simulink model "MOSFET_2L_VSI_SPWM_DDsystem"  (R2023a)
settings: Solver=VariableStepAuto  StartTime=0.0  StopTime=simu.endTime  MaxStep=simu.dt  RelTol=1e-3
undefined symbols (not defined in the file): conv, dev
libraries: WECSim_Lib_PTOSim x2
Description:
  | To be used with Wec-Sim's "Direct Drive Linear Generator" Block. Generator parameters MUST match what was set for simulating the WEC with the associated PTO.
settings Model: Creator=bartonsa  LastModifiedBy=bartonsa

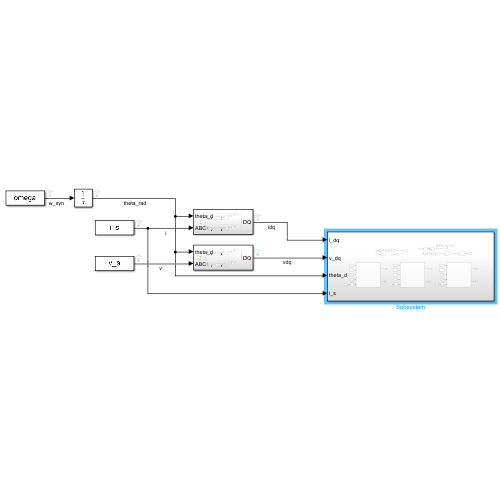
[thumbnail: Simulink's stored preview of the top-level diagram]
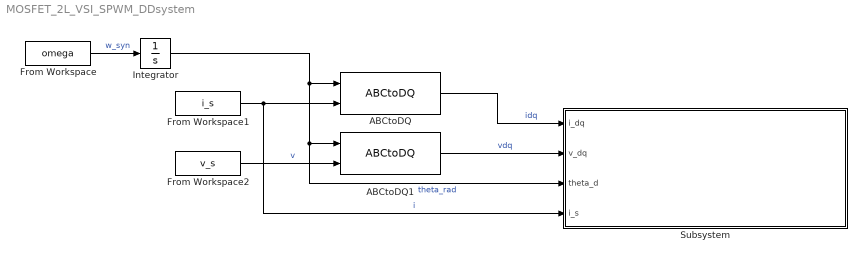
== system MOSFET_2L_VSI_SPWM_DDsystem ==
  ABCtoDQ : WECSim_Lib_PTOSim/Electric/Direct Drive Linear Generator/ABCtoDQ  SystemSampleTime=-1  VariantActivationTime=update diagram  Latency=0  AutoFrameSizeCalculation=off
  ABCtoDQ1 : WECSim_Lib_PTOSim/Electric/Direct Drive Linear Generator/ABCtoDQ  SystemSampleTime=-1  VariantActivationTime=update diagram  Latency=0  AutoFrameSizeCalculation=off
  From Workspace : FromWorkspace  VariableName=omega
  From Workspace1 : FromWorkspace  VariableName=i_s
  From Workspace2 : FromWorkspace  VariableName=v_s
  Integrator : Integrator  WrappedStateLowerValue=0
  Subsystem : Subsystem
  wires:
  ABCtoDQ/1 -> Subsystem/1(i_dq)  "idq"
  ABCtoDQ1/1 -> Subsystem/2(v_dq)  "vdq"
  From Workspace/1 -> Integrator/1  "w_syn"
  Integrator/1 -> Subsystem/3(theta_d), ABCtoDQ1/1, ABCtoDQ/1  "theta_rad"
  From Workspace1/1 -> Subsystem/4(i_s), ABCtoDQ/2  "i"
  From Workspace2/1 -> ABCtoDQ1/2  "v"

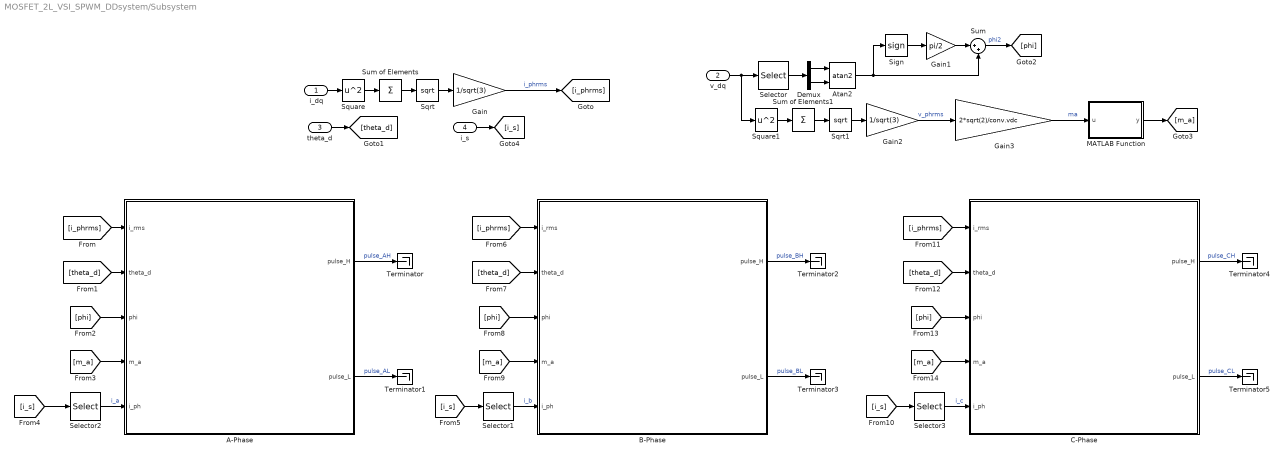
== system MOSFET_2L_VSI_SPWM_DDsystem/Subsystem ==
  i_dq : Inport
  v_dq : Inport  Port=2
  theta_d : Inport  Port=3
  i_s : Inport  Port=4
  A-Phase : Subsystem  AncestorBlock=MPModeling_MOSFETConv_lib/MOSFET 2L VSC/Device 1
      settings: LibrarySourceBlock=MPModeling_MOSFETConv_lib/MOSFET 2L VSC/Device 1
  Atan2 : Trigonometry  Operator=atan2
  B-Phase : Subsystem  AncestorBlock=MPModeling_MOSFETConv_lib/MOSFET 2L VSC/Device 1
      settings: LibrarySourceBlock=MPModeling_MOSFETConv_lib/MOSFET 2L VSC/Device 1
  C-Phase : Subsystem  AncestorBlock=MPModeling_MOSFETConv_lib/MOSFET 2L VSC/Device 1
      settings: LibrarySourceBlock=MPModeling_MOSFETConv_lib/MOSFET 2L VSC/Device 1
  Demux : Demux  Outputs=2
  Gain : Gain  Gain=1/sqrt(3)
  Gain1 : Gain  Gain=pi/2
  Gain2 : Gain  Gain=1/sqrt(3)
  Gain3 : Gain  Gain=2*sqrt(2)/conv.vdc
  MATLAB Function : MATLAB Function  TreatAsAtomicUnit=on
  Selector : Selector  InputPortWidth=2  IndexOptions=Index vector (dialog)  Indices=[2 1]  OutputSizes=1
  Selector1 : Selector  InputPortWidth=3  IndexOptions=Index vector (dialog)  Indices=2  OutputSizes=1
  Selector2 : Selector  InputPortWidth=3  IndexOptions=Index vector (dialog)  Indices=1  OutputSizes=1
  Selector3 : Selector  InputPortWidth=3  IndexOptions=Index vector (dialog)  Indices=3  OutputSizes=1
  Sign : Signum
  Sqrt : Sqrt
  Sqrt1 : Sqrt
  Square : Math  Operator=square
  Square1 : Math  Operator=square
  Sum : Sum  Inputs=|++
  Sum of Elements : Sum  Inputs=+
  Sum of Elements1 : Sum  Inputs=+
  Terminator{,1..5} (6 alike) : Terminator
  wires:
  Sum of Elements/1 -> Sqrt/1
  v_dq/1 -> Selector/1, Square1/1
  Gain/1 -> [i_phrms]  "i_phrms"
  i_dq/1 -> Square/1
  Square/1 -> Sum of Elements/1
  theta_d/1 -> [theta_d]
  Selector/1 -> Demux/1
  Sqrt/1 -> Gain/1
  A-Phase/1(pulse_H) -> Terminator/1  "pulse_AH"
  Demux/1 -> Atan2/1
  Demux/2 -> Atan2/2
  Atan2/1 -> Sum/2, Sign/1
  Square1/1 -> Sum of Elements1/1
  Sqrt1/1 -> Gain2/1
  Sum of Elements1/1 -> Sqrt1/1
  Gain2/1 -> Gain3/1  "v_phrms"
  Gain3/1 -> MATLAB Function/1(u)  "ma"
  i_s/1 -> [i_s]
  Selector2/1 -> A-Phase/5(i_ph)  "i_a"
  A-Phase/2(pulse_L) -> Terminator1/1  "pulse_AL"
  [i_phrms] -> A-Phase/1(i_rms)
  [theta_d] -> A-Phase/2(theta_d)
  [phi] -> A-Phase/3(phi)
  [m_a] -> A-Phase/4(m_a)
  [i_s] -> Selector2/1
  Selector1/1 -> B-Phase/5(i_ph)  "i_b"
  [i_s] -> Selector1/1
  [i_phrms] -> B-Phase/1(i_rms)
  [theta_d] -> B-Phase/2(theta_d)
  [phi] -> B-Phase/3(phi)
  [m_a] -> B-Phase/4(m_a)
  B-Phase/2(pulse_L) -> Terminator3/1  "pulse_BL"
  B-Phase/1(pulse_H) -> Terminator2/1  "pulse_BH"
  [phi] -> C-Phase/3(phi)
  C-Phase/2(pulse_L) -> Terminator5/1  "pulse_CL"
  [theta_d] -> C-Phase/2(theta_d)
  [i_phrms] -> C-Phase/1(i_rms)
  C-Phase/1(pulse_H) -> Terminator4/1  "pulse_CH"
  Selector3/1 -> C-Phase/5(i_ph)  "i_c"
  [i_s] -> Selector3/1
  [m_a] -> C-Phase/4(m_a)
  MATLAB Function/1(y) -> [m_a]
  Sign/1 -> Gain1/1
  Gain1/1 -> Sum/1
  Sum/1 -> [phi]  "phi2"

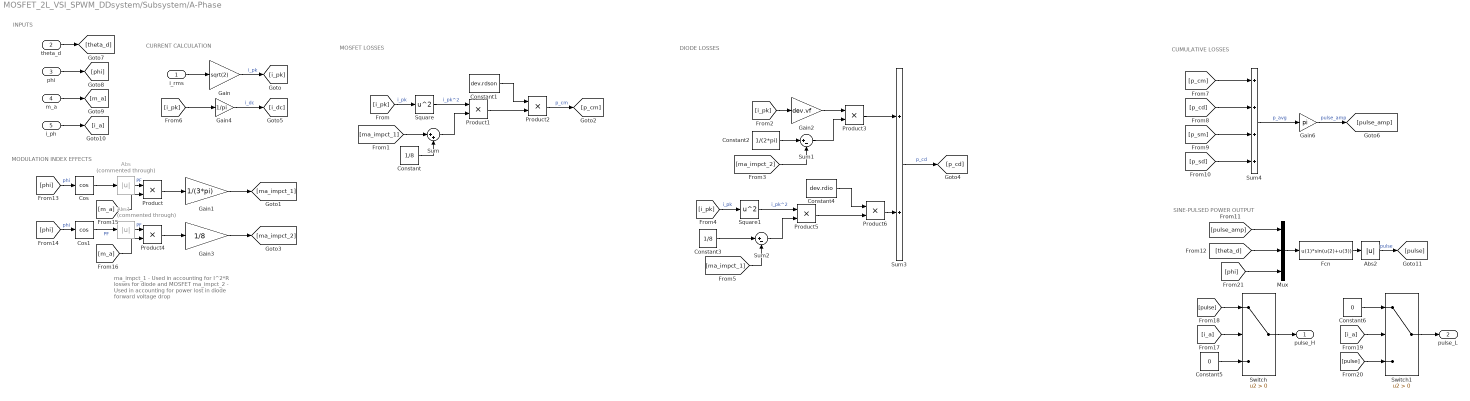
== system MOSFET_2L_VSI_SPWM_DDsystem/Subsystem/A-Phase ==
  note: INPUTS
  note: CURRENT CALCULATION
  note: SINE-PULSED POWER OUTPUT
  note: MODULATION INDEX EFFECTS
  note: ma_impct_1 - Used in accounting for I^2*R losses for diode and MOSFET
      |
      | ma_impct_2 - Used in accounting for power lost in diode forward voltage drop
  note: MOSFET LOSSES
  note: DIODE LOSSES
  note: CUMULATIVE LOSSES
  i_rms : Inport
  theta_d : Inport  Port=2
  phi : Inport  Port=3
  m_a : Inport  Port=4
  i_ph : Inport  Port=5
  Abs : Abs  Commented=through  SaturateOnIntegerOverflow=off
  Abs1 : Abs  Commented=through  SaturateOnIntegerOverflow=off
  Abs2 : Abs  SaturateOnIntegerOverflow=off
  Constant : Constant  Value=1/8
  Constant1 : Constant  Value=dev.rdson
  Constant2 : Constant  Value=1/(2*pi)
  Constant3 : Constant  Value=1/8
  Constant4 : Constant  Value=dev.rdio
  Constant5 : Constant  Value=0
  Constant6 : Constant  Value=0
  Cos : Trigonometry  Operator=cos
  Cos1 : Trigonometry  Operator=cos
  Fcn : Fcn  Expr=u(1)*sin(u(2)+u(3))
  Gain : Gain  Gain=sqrt(2)
  Gain1 : Gain  Gain=1/(3*pi)
  Gain2 : Gain  Gain=dev.vf
  Gain3 : Gain  Gain=1/8
  Gain4 : Gain  Gain=1/pi
  Gain6 : Gain  Gain=pi
  Mux : Mux  Inputs=3
  Product{,1..6} (7 alike) : Product
  Square : Math  Operator=square
  Square1 : Math  Operator=square
  Sum : Sum  Inputs=|++
  Sum1 : Sum  Inputs=|+-
  Sum2 : Sum  Inputs=|+-
  Sum3 : Sum
  Sum4 : Sum  Inputs=++++
  Switch : Switch  Criteria=u2 > Threshold  SaturateOnIntegerOverflow=off  InputSameDT=off
  Switch1 : Switch  Criteria=u2 > Threshold  SaturateOnIntegerOverflow=off  InputSameDT=off
  pulse_H : Outport
  pulse_L : Outport  Port=2
  wires:
  Mux/1 -> Fcn/1
  m_a/1 -> [m_a]
  phi/1 -> [phi]
  Abs2/1 -> [pulse]  "pulse"
  theta_d/1 -> [theta_d]
  [phi] -> Cos/1  "phi"
  Sum2/1 -> Product5/2
  [ma_impct_1] -> Sum2/2
  Constant3/1 -> Sum2/1
  Square1/1 -> Product5/1  "i_pk^2"
  Constant2/1 -> Sum1/1
  Gain2/1 -> Product3/1
  Cos1/1 -> Abs1/1  "PF"
  Gain3/1 -> [ma_impct_2]
  [ma_impct_1] -> Sum/1
  Fcn/1 -> Abs2/1
  Sum4/1 -> Gain6/1  "p_avg"
  [p_sd] -> Sum4/4
  Product6/1 -> Sum3/2
  [p_cm] -> Sum4/1
  [p_cd] -> Sum4/2
  [phi] -> Cos1/1  "phi"
  Gain4/1 -> [i_dc]  "i_dc"
  Constant4/1 -> Product6/1
  [i_pk] -> Gain2/1
  Constant1/1 -> Product2/1
  Product3/1 -> Sum3/1
  [i_pk] -> Gain4/1
  Product2/1 -> [p_cm]  "p_cm"
  Product4/1 -> Gain3/1
  Sum1/1 -> Product3/2
  i_rms/1 -> Gain/1
  [ma_impct_2] -> Sum1/2
  Square/1 -> Product1/1  "i_pk^2"
  Constant/1 -> Sum/2
  Gain/1 -> [i_pk]  "i_pk"
  [i_pk] -> Square1/1  "i_pk"
  Product5/1 -> Product6/2
  Cos/1 -> Abs/1
  Product1/1 -> Product2/2
  Sum3/1 -> [p_cd]  "p_cd"
  [i_pk] -> Square/1  "i_pk"
  Gain1/1 -> [ma_impct_1]
  [p_sm] -> Sum4/3
  [pulse_amp] -> Mux/1
  Sum/1 -> Product1/2
  Product/1 -> Gain1/1
  Abs/1 -> Product/1  "PF"
  Abs1/1 -> Product4/1  "PF"
  [m_a] -> Product/2
  [m_a] -> Product4/2
  [theta_d] -> Mux/2
  Switch/1 -> pulse_H/1
  [i_a] -> Switch/2
  Constant5/1 -> Switch/3
  Gain6/1 -> [pulse_amp]  "pulse_amp"
  i_ph/1 -> [i_a]
  [pulse] -> Switch/1
  Switch1/1 -> pulse_L/1
  [i_a] -> Switch1/2
  Constant6/1 -> Switch1/1
  [pulse] -> Switch1/3
  [phi] -> Mux/3

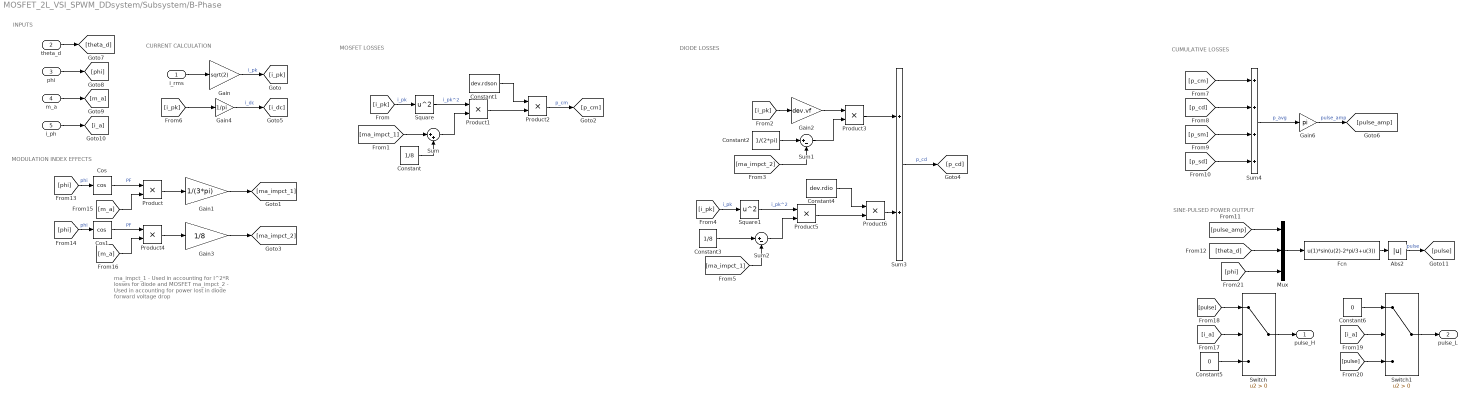
== system MOSFET_2L_VSI_SPWM_DDsystem/Subsystem/B-Phase ==
  note: INPUTS
  note: CURRENT CALCULATION
  note: SINE-PULSED POWER OUTPUT
  note: MODULATION INDEX EFFECTS
  note: ma_impct_1 - Used in accounting for I^2*R losses for diode and MOSFET
      |
      | ma_impct_2 - Used in accounting for power lost in diode forward voltage drop
  note: MOSFET LOSSES
  note: DIODE LOSSES
  note: CUMULATIVE LOSSES
  i_rms : Inport
  theta_d : Inport  Port=2
  phi : Inport  Port=3
  m_a : Inport  Port=4
  i_ph : Inport  Port=5
  Abs2 : Abs  SaturateOnIntegerOverflow=off
  Constant : Constant  Value=1/8
  Constant1 : Constant  Value=dev.rdson
  Constant2 : Constant  Value=1/(2*pi)
  Constant3 : Constant  Value=1/8
  Constant4 : Constant  Value=dev.rdio
  Constant5 : Constant  Value=0
  Constant6 : Constant  Value=0
  Cos : Trigonometry  Operator=cos
  Cos1 : Trigonometry  Operator=cos
  Fcn : Fcn  Expr=u(1)*sin(u(2)-2*pi/3+u(3))
  Gain : Gain  Gain=sqrt(2)
  Gain1 : Gain  Gain=1/(3*pi)
  Gain2 : Gain  Gain=dev.vf
  Gain3 : Gain  Gain=1/8
  Gain4 : Gain  Gain=1/pi
  Gain6 : Gain  Gain=pi
  Mux : Mux  Inputs=3
  Product{,1..6} (7 alike) : Product
  Square : Math  Operator=square
  Square1 : Math  Operator=square
  Sum : Sum  Inputs=|++
  Sum1 : Sum  Inputs=|+-
  Sum2 : Sum  Inputs=|+-
  Sum3 : Sum
  Sum4 : Sum  Inputs=++++
  Switch : Switch  Criteria=u2 > Threshold  SaturateOnIntegerOverflow=off  InputSameDT=off
  Switch1 : Switch  Criteria=u2 > Threshold  SaturateOnIntegerOverflow=off  InputSameDT=off
  pulse_H : Outport
  pulse_L : Outport  Port=2
  wires:
  Mux/1 -> Fcn/1
  m_a/1 -> [m_a]
  phi/1 -> [phi]
  Abs2/1 -> [pulse]  "pulse"
  theta_d/1 -> [theta_d]
  [phi] -> Cos/1  "phi"
  Sum2/1 -> Product5/2
  [ma_impct_1] -> Sum2/2
  Constant3/1 -> Sum2/1
  Square1/1 -> Product5/1  "i_pk^2"
  Constant2/1 -> Sum1/1
  Gain2/1 -> Product3/1
  Gain3/1 -> [ma_impct_2]
  [ma_impct_1] -> Sum/1
  Fcn/1 -> Abs2/1
  Sum4/1 -> Gain6/1  "p_avg"
  [p_sd] -> Sum4/4
  Product6/1 -> Sum3/2
  [p_cm] -> Sum4/1
  [p_cd] -> Sum4/2
  [phi] -> Cos1/1  "phi"
  Gain4/1 -> [i_dc]  "i_dc"
  Constant4/1 -> Product6/1
  [i_pk] -> Gain2/1
  Constant1/1 -> Product2/1
  Product3/1 -> Sum3/1
  [i_pk] -> Gain4/1
  Product2/1 -> [p_cm]  "p_cm"
  Product4/1 -> Gain3/1
  Sum1/1 -> Product3/2
  i_rms/1 -> Gain/1
  [ma_impct_2] -> Sum1/2
  Square/1 -> Product1/1  "i_pk^2"
  Constant/1 -> Sum/2
  Gain/1 -> [i_pk]  "i_pk"
  [i_pk] -> Square1/1  "i_pk"
  Product5/1 -> Product6/2
  Product1/1 -> Product2/2
  Sum3/1 -> [p_cd]  "p_cd"
  [i_pk] -> Square/1  "i_pk"
  Gain1/1 -> [ma_impct_1]
  [p_sm] -> Sum4/3
  [pulse_amp] -> Mux/1
  Sum/1 -> Product1/2
  Product/1 -> Gain1/1
  Cos/1 -> Product/1  "PF"
  Cos1/1 -> Product4/1  "PF"
  [m_a] -> Product/2
  [m_a] -> Product4/2
  [theta_d] -> Mux/2
  Switch/1 -> pulse_H/1
  [i_a] -> Switch/2
  Constant5/1 -> Switch/3
  Gain6/1 -> [pulse_amp]  "pulse_amp"
  i_ph/1 -> [i_a]
  [pulse] -> Switch/1
  Switch1/1 -> pulse_L/1
  [i_a] -> Switch1/2
  Constant6/1 -> Switch1/1
  [pulse] -> Switch1/3
  [phi] -> Mux/3

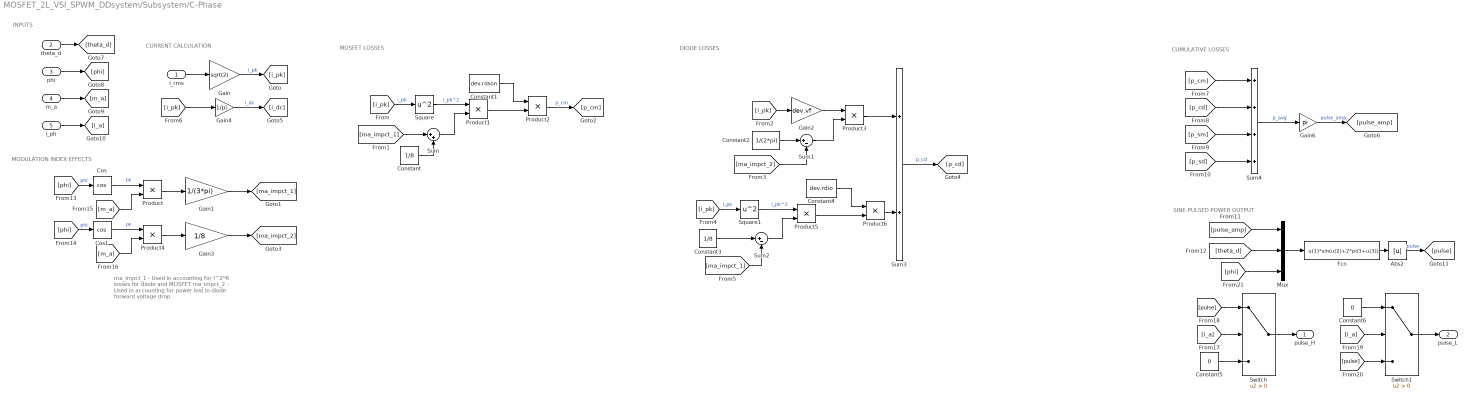
== system MOSFET_2L_VSI_SPWM_DDsystem/Subsystem/C-Phase ==
  note: INPUTS
  note: CURRENT CALCULATION
  note: SINE-PULSED POWER OUTPUT
  note: MODULATION INDEX EFFECTS
  note: ma_impct_1 - Used in accounting for I^2*R losses for diode and MOSFET
      |
      | ma_impct_2 - Used in accounting for power lost in diode forward voltage drop
  note: MOSFET LOSSES
  note: DIODE LOSSES
  note: CUMULATIVE LOSSES
  i_rms : Inport
  theta_d : Inport  Port=2
  phi : Inport  Port=3
  m_a : Inport  Port=4
  i_ph : Inport  Port=5
  Abs2 : Abs  SaturateOnIntegerOverflow=off
  Constant : Constant  Value=1/8
  Constant1 : Constant  Value=dev.rdson
  Constant2 : Constant  Value=1/(2*pi)
  Constant3 : Constant  Value=1/8
  Constant4 : Constant  Value=dev.rdio
  Constant5 : Constant  Value=0
  Constant6 : Constant  Value=0
  Cos : Trigonometry  Operator=cos
  Cos1 : Trigonometry  Operator=cos
  Fcn : Fcn  Expr=u(1)*sin(u(2)+2*pi/3+u(3))
  Gain : Gain  Gain=sqrt(2)
  Gain1 : Gain  Gain=1/(3*pi)
  Gain2 : Gain  Gain=dev.vf
  Gain3 : Gain  Gain=1/8
  Gain4 : Gain  Gain=1/pi
  Gain6 : Gain  Gain=pi
  Mux : Mux  Inputs=3
  Product{,1..6} (7 alike) : Product
  Square : Math  Operator=square
  Square1 : Math  Operator=square
  Sum : Sum  Inputs=|++
  Sum1 : Sum  Inputs=|+-
  Sum2 : Sum  Inputs=|+-
  Sum3 : Sum
  Sum4 : Sum  Inputs=++++
  Switch : Switch  Criteria=u2 > Threshold  SaturateOnIntegerOverflow=off  InputSameDT=off
  Switch1 : Switch  Criteria=u2 > Threshold  SaturateOnIntegerOverflow=off  InputSameDT=off
  pulse_H : Outport
  pulse_L : Outport  Port=2
  wires:
  Mux/1 -> Fcn/1
  m_a/1 -> [m_a]
  phi/1 -> [phi]
  Abs2/1 -> [pulse]  "pulse"
  theta_d/1 -> [theta_d]
  [phi] -> Cos/1  "phi"
  Sum2/1 -> Product5/2
  [ma_impct_1] -> Sum2/2
  Constant3/1 -> Sum2/1
  Square1/1 -> Product5/1  "i_pk^2"
  Constant2/1 -> Sum1/1
  Gain2/1 -> Product3/1
  Gain3/1 -> [ma_impct_2]
  [ma_impct_1] -> Sum/1
  Fcn/1 -> Abs2/1
  Sum4/1 -> Gain6/1  "p_avg"
  [p_sd] -> Sum4/4
  Product6/1 -> Sum3/2
  [p_cm] -> Sum4/1
  [p_cd] -> Sum4/2
  [phi] -> Cos1/1  "phi"
  Gain4/1 -> [i_dc]  "i_dc"
  Constant4/1 -> Product6/1
  [i_pk] -> Gain2/1
  Constant1/1 -> Product2/1
  Product3/1 -> Sum3/1
  [i_pk] -> Gain4/1
  Product2/1 -> [p_cm]  "p_cm"
  Product4/1 -> Gain3/1
  Sum1/1 -> Product3/2
  i_rms/1 -> Gain/1
  [ma_impct_2] -> Sum1/2
  Square/1 -> Product1/1  "i_pk^2"
  Constant/1 -> Sum/2
  Gain/1 -> [i_pk]  "i_pk"
  [i_pk] -> Square1/1  "i_pk"
  Product5/1 -> Product6/2
  Product1/1 -> Product2/2
  Sum3/1 -> [p_cd]  "p_cd"
  [i_pk] -> Square/1  "i_pk"
  Gain1/1 -> [ma_impct_1]
  [p_sm] -> Sum4/3
  [pulse_amp] -> Mux/1
  Sum/1 -> Product1/2
  Product/1 -> Gain1/1
  Cos/1 -> Product/1  "PF"
  Cos1/1 -> Product4/1  "PF"
  [m_a] -> Product/2
  [m_a] -> Product4/2
  [theta_d] -> Mux/2
  Switch/1 -> pulse_H/1
  [i_a] -> Switch/2
  Constant5/1 -> Switch/3
  Gain6/1 -> [pulse_amp]  "pulse_amp"
  i_ph/1 -> [i_a]
  [pulse] -> Switch/1
  Switch1/1 -> pulse_L/1
  [i_a] -> Switch1/2
  Constant6/1 -> Switch1/1
  [pulse] -> Switch1/3
  [phi] -> Mux/3

== matlab function MOSFET_2L_VSI_SPWM_DDsystem/Subsystem/MATLAB Function ==
  data: u input; y output
function y = checkMa(u)

if u > 1
    error('Modulation index (ma) greater than 1.');
end

y = u;
